simulink subsystem "FrequencyIn"  (R2024a)
settings: Solver=VariableStepAuto  StartTime=0.0  StopTime=10.0  RelTol=1e-3
undefined symbols (not defined in the file or in its folder): xtones
settings Model: Creator=dfurodet  LastModifiedBy=david
settings RTWCC: GPUComputeCapability=3.5

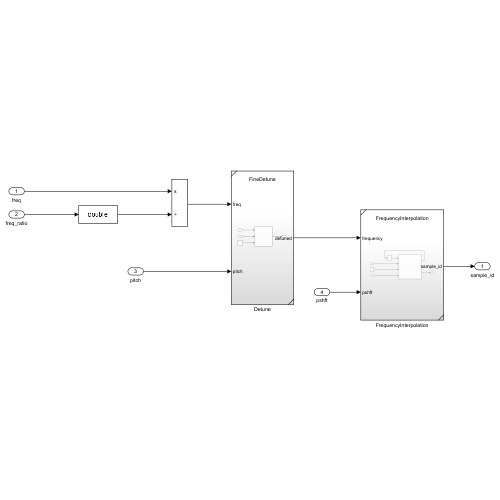
[thumbnail: Simulink's stored preview of the top-level diagram]
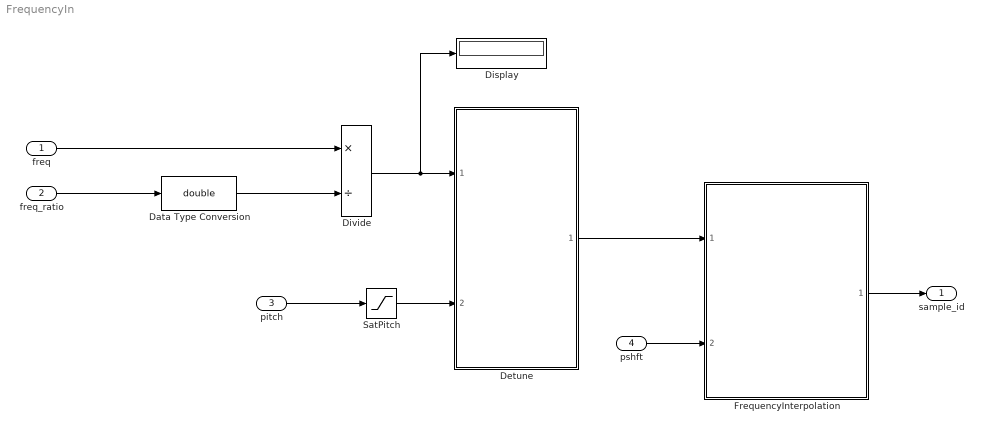
== system FrequencyIn ==
  freq : Inport
  freq_ratio : Inport  Port=2
  pitch : Inport  Port=3
  pshft : Inport  Port=4
  Data Type Conversion : DataTypeConversion  OutDataTypeStr=double  SaturateOnIntegerOverflow=off  RndMeth=Floor
  Detune : Subsystem  ReferencedSubsystem=FineDetune
  Display : Display
  Divide : Product  Inputs=*/
  FrequencyInterpolation : Subsystem  ReferencedSubsystem=FrequencyInterpolation
  SatPitch : Saturate  UpperLimit=xtones  LowerLimit=0
  sample_id : Outport
  wires:
  FrequencyInterpolation/1 -> sample_id/1
  pshft/1 -> FrequencyInterpolation/2
  pitch/1 -> SatPitch/1
  Detune/1 -> FrequencyInterpolation/1
  freq/1 -> Divide/1
  Divide/1 -> Detune/1, Display/1
  freq_ratio/1 -> Data Type Conversion/1
  Data Type Conversion/1 -> Divide/2
  SatPitch/1 -> Detune/2
